simulink model "aircraft_simulation"  (R2015a)
settings: Solver=ode45  StartTime=0.0  StopTime=10000  RelTol=1e-3
values from neighbouring files (symbols this model uses):
  aircraft_parameters =     [TestVariablesLab3.mat]
  control_surfaces_trim = [5*(pi/180) 2*(pi/180) -13*(pi/180) .3]    [RunSimLab3.m]
undefined symbols (not defined in the file or in its folder): drawAircraft, PlotStateVariables, pts, S_AeroForcesAndMoments
libraries: simulink x4, aerolib6dof2 x1
settings Model: CovSFcnEnable=off  Creator=beard  LastModifiedBy=dylanrichards
settings DataIOCC: SignalLoggingSaveFormat=ModelDataLogs
settings OptimizationCC: ExpressionDepthLimit=2147483647  InitFltsAndDblsToZero=on
settings DebuggingCC: UnderspecifiedInitializationDetection=Classic  MergeDetectMultiDrivingBlocksExec=none  SolverPrmCheckMsg=warning  FcnCallInpInsideContextMsg=UseLocalSettings  StateNameClashWarn=warning
settings GRTTargetCC: CombineOutputUpdateFcns=off  GRTInterface=on

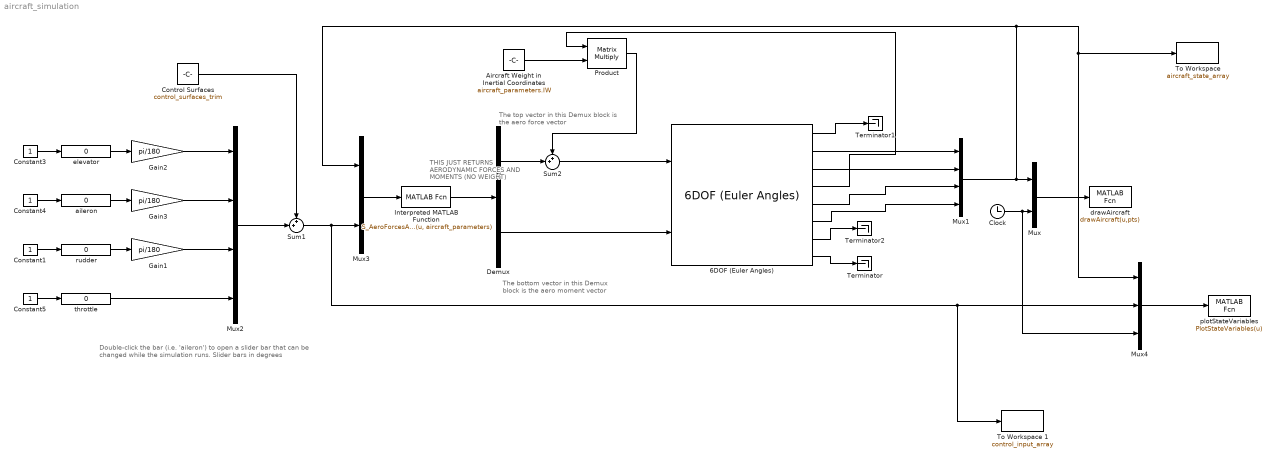
== system aircraft_simulation ==
  note: Double-click the bar (i.e. 'aileron') to open a slider bar that
      | can be changed while the simulation runs. Slider bars in degrees
  note: THIS JUST RETURNS AERODYNAMIC
      | FORCES AND MOMENTS (NO WEIGHT)
  note: The top vector in this Demux block
      |  is the aero force vector
  note: The bottom vector in this Demux
      | block is the aero moment vector
  6DOF (Euler Angles) : aerolib6dof2/6DOF (Euler Angles)  units=Metric (MKS)  mtype=Fixed  rep=Euler Angles  xme_0=position_inertial  Vm_0=velocity_body  eul_0=euler_angles  pm_0=omega_body  mass_0=aircraft_parameters.m  mass_e=0.5  mass_f=2.0  inertia=inertia_matrix  inertia_e=eye(3)  inertia_f=2*eye(3)  k_quat=1.0  vre_flag=on
  Aircraft Weight in Inertial Coordinates : Constant  Value=aircraft_parameters.IW
  Clock : Clock
  Constant{1,3..5} (4 alike) : Constant
  Control Surfaces : Constant  Value=control_surfaces_trim
  Demux : Demux  Outputs=2
  Gain1 : Gain  Gain=pi/180
  Gain2 : Gain  Gain=pi/180
  Gain3 : Gain  Gain=pi/180
  Interpreted MATLAB Function : MATLABFcn  MATLABFcn=S_AeroForcesAndMoments(u, aircraft_parameters)  OutputDimensions=6
  Mux : Mux  Inputs=2
  Mux1 : Mux
  Mux2 : Mux
  Mux3 : Mux  Inputs=2
  Mux4 : Mux  Inputs=3
  Product : Product  Multiplication=Matrix(*)
  Sum1 : Sum  Inputs=++|
  Sum2 : Sum  Inputs=++|
  Terminator : Terminator
  Terminator1 : Terminator
  Terminator2 : Terminator
  To Workspace : ToWorkspace  VariableName=aircraft_state_array  SaveFormat=Timeseries  SampleTime=-1
  To Workspace 1 : ToWorkspace  VariableName=control_input_array  SaveFormat=Timeseries  SampleTime=-1
  aileron : simulink/Math Operations/Slider Gain  low=-180  gain=0  high=180
  drawAircraft : MATLABFcn  MATLABFcn=drawAircraft(u,pts)  OutputDimensions=0
  elevator : simulink/Math Operations/Slider Gain  low=-180  gain=0  high=180
  plotStateVariables : MATLABFcn  MATLABFcn=PlotStateVariables(u)  OutputDimensions=0
  rudder : simulink/Math Operations/Slider Gain  low=-180  gain=0  high=180
  throttle : simulink/Math Operations/Slider Gain  low=0  gain=0  high=1
  wires:
  Constant3/1 -> elevator/1
  elevator/1 -> Gain2/1
  Constant4/1 -> aileron/1
  Mux/1 -> drawAircraft/1
  Clock/1 -> Mux4/3, Mux/2
  aileron/1 -> Gain3/1
  rudder/1 -> Gain1/1
  Constant1/1 -> rudder/1
  Gain2/1 -> Mux2/1
  Gain3/1 -> Mux2/2
  Gain1/1 -> Mux2/3
  Mux1/1 -> To Workspace/1, Mux4/1, Mux3/1, Mux/1
  Constant5/1 -> throttle/1
  throttle/1 -> Mux2/4
  Mux3/1 -> Interpreted MATLAB Function/1
  Interpreted MATLAB Function/1 -> Demux/1
  Sum1/1 -> To Workspace 1/1, Mux4/2, Mux3/2
  Mux4/1 -> plotStateVariables/1
  Mux2/1 -> Sum1/2
  Control Surfaces/1 -> Sum1/1
  6DOF (Euler Angles)/1 -> Terminator1/1
  6DOF (Euler Angles)/7 -> Terminator2/1
  6DOF (Euler Angles)/8 -> Terminator/1
  6DOF (Euler Angles)/2 -> Mux1/1
  6DOF (Euler Angles)/3 -> Mux1/2
  6DOF (Euler Angles)/6 -> Mux1/4
  6DOF (Euler Angles)/5 -> Mux1/3
  6DOF (Euler Angles)/4 -> Product/1
  Aircraft Weight in Inertial Coordinates/1 -> Product/2
  Product/1 -> Sum2/1
  Demux/1 -> Sum2/2
  Sum2/1 -> 6DOF (Euler Angles)/1
  Demux/2 -> 6DOF (Euler Angles)/2
